simulink model "Kurs"  (R2024a)
settings: Solver=ode1  StartTime=0.0  StopTime=1.2  FixedStep=0.000001  RelTol=1e-3
InitFcn:
  | Kpr = 56;
  | Tpr = 0.002;
  | Rya = 1.78;
  | Tya = 0.16;
  | c = 0.56;
  | J = 0.05;
  | Kot = 0.054;
  | Koc = 0.09;
  | T1 = 0.0013;
  | T2 = 0.0165;
  | T4 = 0.207;
  | K1 = 6.74;
  | K2 = 3.12;
  | K3 = 0.874;
  | X1max = 3;
  | Y2max = 250;
  | Y4max = 90;
  | Z = 17;
  | treg = 0.001;
  | toy = 0.0001;
undefined symbols (not defined in the file or in its folder): Kaw, tre
libraries: slpidlib x5
(part 2 of 2)

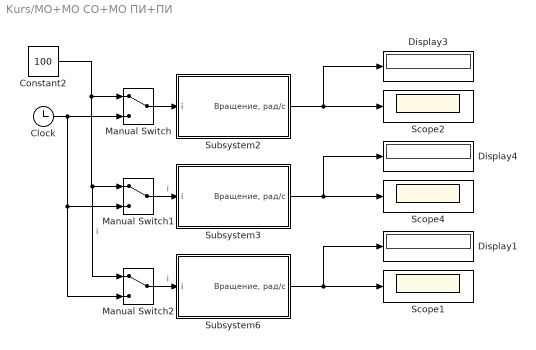
== system Kurs/МО+МО СО+МО ПИ+ПИ ==
  Clock : Clock
  Constant2 : Constant  Value=100
  Display1 : Display
  Display3 : Display
  Display4 : Display
  Manual Switch : ManualSwitch
  Manual Switch1 : ManualSwitch
  Manual Switch2 : ManualSwitch
  Scope1 : Scope
  Scope2 : Scope
  Scope4 : Scope
  Subsystem2 : Subsystem
      mask Display: disp('МО+МО');
  Subsystem3 : Subsystem
      mask Display: disp('СО+МО');
  Subsystem6 : Subsystem  mask{Kpr=Kpr, Tpr=Tpr, Rya=Rya, Tya=Tya, Cm=c, Ce=c, Kot=Kot, Koc=Koc, treg=0.001, toy=Tpr / 100}
      mask prompts: Kpr "Коэффициент усиления преобразователя"; Tpr "Постоянная времени преобразователя"; Rya "Коэффициент усиления тока (1/Rya)"; Tya "Постоянная времени тока"; Cm "Постоянный конструктивный коэффициент (коэффициент связи)"; Ce "Постоянный конструктивный коэффициент (u = Ce*w)"; Kot "Коэффициент обратной связи тока"; Koc "Коэффициент обратной связи угловой скорости"; treg "Шаг дискретизации регуляторов"; toy "Шаг дискретизации ОУ"
      mask Display: disp('ПИ+ПИ');
  wires:
  Subsystem2/1("Вращение, рад/с") -> Display3/1, Scope2/1
  Constant2/1 -> Manual Switch2/1, Manual Switch1/1, Manual Switch/1  "i"
  Subsystem3/1("Вращение, рад/с") -> Display4/1, Scope4/1
  Manual Switch2/1 -> Subsystem6/1(i)  "i"
  Clock/1 -> Manual Switch2/2, Manual Switch1/2, Manual Switch/2
  Subsystem6/1("Вращение, рад/с") -> Display1/1, Scope1/1
  Manual Switch1/1 -> Subsystem3/1(i)  "i"
  Manual Switch/1 -> Subsystem2/1(i)

== system Kurs/МО СО ПИ-регулятор/Subsystem ==
  i : Inport
  1/(rя*(Ts+1)) : TransferFcn  Numerator=[1/Rya]  Denominator=[Tya 1]
  Display : Display
  Gain : Gain  Gain=Tya*Rya/(2*Kpr*Tpr)
  Gain1 : Gain  Gain=1/Tya
  Integrator : Integrator
  Sum : Sum  Inputs=|++
  Sum1 : Sum  Inputs=|+-
  kt/(Ts+1) : TransferFcn  Numerator=[Kpr]  Denominator=[Tpr 1]
  "Ток, А" : Outport
  wires:
  i/1 -> Sum1/1
  kt/(Ts+1)/1 -> 1/(rя*(Ts+1))/1
  Gain1/1 -> Integrator/1
  Gain/1 -> Gain1/1, Display/1, Sum/1
  Integrator/1 -> Sum/2
  1/(rя*(Ts+1))/1 -> "Ток, А"/1, Sum1/2  "Ток, А"
  Sum/1 -> kt/(Ts+1)/1  "U"
  Sum1/1 -> Gain/1  "e(i)"

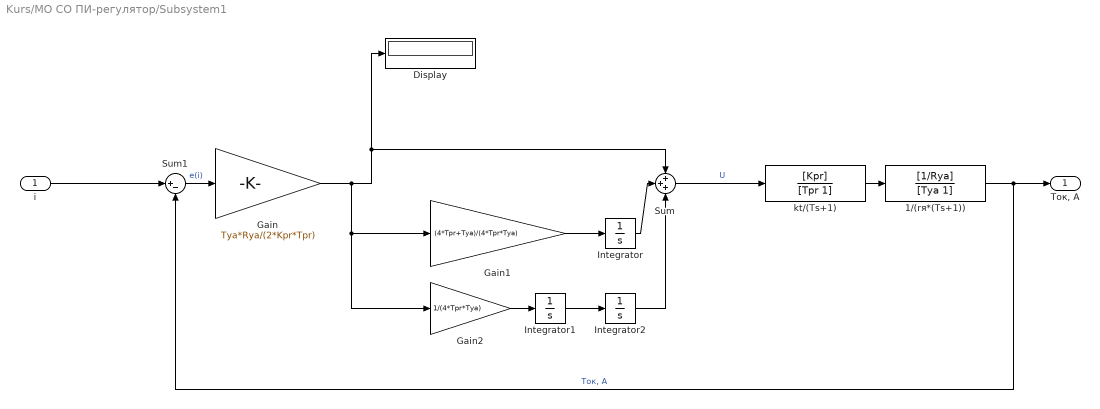
== system Kurs/МО СО ПИ-регулятор/Subsystem1 ==
  i : Inport
  1/(rя*(Ts+1)) : TransferFcn  Numerator=[1/Rya]  Denominator=[Tya 1]
  Display : Display
  Gain : Gain  Gain=Tya*Rya/(2*Kpr*Tpr)
  Gain1 : Gain  Gain=(4*Tpr+Tya)/(4*Tpr*Tya)
  Gain2 : Gain  Gain=1/(4*Tpr*Tya)
  Integrator : Integrator
  Integrator1 : Integrator
  Integrator2 : Integrator
  Sum : Sum  Inputs=+++
  Sum1 : Sum  Inputs=|+-
  kt/(Ts+1) : TransferFcn  Numerator=[Kpr]  Denominator=[Tpr 1]
  "Ток, А" : Outport
  wires:
  i/1 -> Sum1/1
  kt/(Ts+1)/1 -> 1/(rя*(Ts+1))/1
  Gain1/1 -> Integrator/1
  Gain/1 -> Gain2/1, Gain1/1, Display/1, Sum/1
  Integrator/1 -> Sum/2
  1/(rя*(Ts+1))/1 -> "Ток, А"/1, Sum1/2  "Ток, А"
  Sum/1 -> kt/(Ts+1)/1  "U"
  Sum1/1 -> Gain/1  "e(i)"
  Gain2/1 -> Integrator1/1
  Integrator1/1 -> Integrator2/1
  Integrator2/1 -> Sum/3

== system Kurs/МО СО ПИ-регулятор/Subsystem5 ==
  i0(t) : Inport
  1/(rя*(Ts+1)) : TransferFcn  Numerator=[1/Rya]  Denominator=[Tya 1]
  PID Controller9 : slpidlib/PID Controller  Controller=PI  Form=Parallel  TimeDomain=Continuous-time  UseExternalTs=off  SampleTime=treg  IntegratorMethod=Forward Euler  FilterMethod=Forward Euler  ControllerParametersSource=internal  P=0.186679429770122  I=1.09570846442157  UseKiTs=off  D=-544.981619005016  UseExternalDerivativeSource=off  N=0.000737427491300299  UseFilter=on  TunerSelectOption=Transfer Function Based (PID Tuner App)  InitialConditionSource=internal  InitialConditionForIntegrator=0  InitialConditionForFilter=0  DifferentiatorICPrevScaledInput=0  ExternalReset=none  TrackingMode=off  Kt=1  LimitOutput=off  SatLimitsSource=internal  UpperSaturationLimit=12  LowerSaturationLimit=-12  LinearizeAsGain=on  AntiWindupMode=none  Kb=1  LimitIntegrator=off  UpperIntegratorSaturationLimit=inf  LowerIntegratorSaturationLimit=-inf  POutMin=[]  POutMax=[]  IOutMin=[]  IOutMax=[]  DOutMin=[]  DOutMax=[]  NOutMin=[]  NOutMax=[]  SumOutMin=[]  SumOutMax=[]  SaturationOutMin=[]  SaturationOutMax=[]  PParamMin=[]  PParamMax=[]  IParamMin=[]  IParamMax=[]  DParamMin=[]  DParamMax=[]  NParamMin=[]  NParamMax=[]  KbParamMin=[]  KbParamMax=[]  KtParamMin=[]  KtParamMax=[]  KbOutMin=[]  KbOutMax=[]  KtOutMin=[]  KtOutMax=[]  IntegratorOutMin=[]  IntegratorOutMax=[]  FilterOutMin=[]  FilterOutMax=[]  SumI1OutMin=[]  SumI1OutMax=[]  SumI2OutMin=[]  SumI2OutMax=[]  SumI3OutMin=[]  SumI3OutMax=[]  SumI4OutMin=[]  SumI4OutMax=[]  SumDOutMin=[]  SumDOutMax=[]  DifferentiatorOutMin=[]  DifferentiatorOutMax=[]  FilterDiffOutCoefMin=[]  FilterDiffOutCoefMax=[]  ReciprocalOutMin=[]  ReciprocalOutMax=[]  SumDenOutMin=[]  SumDenOutMax=[]  SumNumOutMin=[]  SumNumOutMax=[]  DivideOutMin=[]  DivideOutMax=[]  UdiffTsProdOutMin=[]  UdiffTsProdOutMax=[]  NTsProdOutMin=[]  NTsProdOutMax=[]  UintegralTsProdOutMin=[]  UintegralTsProdOutMax=[]  UngainTsProdOutMin=[]  UngainTsProdOutMax=[]  ClampingZeroOutDataTypeStr=Inherit: Inherit via back propagation  ClampingZeroOutMin=[]  ClampingZeroOutMax=[]  FilterDenConstantOutDataTypeStr=Inherit: Inherit via back propagation  FilterDenConstantOutMin=[]  FilterDenConstantOutMax=[]  PCopyOutDataTypeStr=Inherit: Inherit via back propagation  PCopyOutMin=[]  PCopyOutMax=[]  NCopyOutDataTypeStr=Inherit: Inherit via back propagation  NCopyOutMin=[]  NCopyOutMax=[]  IntegratorContinuousStateAttributes=''  IntegratorStateMustResolveToSignalObject=off  IntegratorRTWStateStorageClass=Auto  FilterContinuousStateAttributes=''  FilterStateMustResolveToSignalObject=off  FilterRTWStateStorageClass=Auto  ParallelPVariant=InternalParameters  IdealPVariant=Disabled  IVariant=InternalParameters  DVariant=Disabled  IntegratorVariant=Continuous  SatVariant=Disabled  AWVariant=Passthrough  PCopyVariant=Disabled  TRVariant=Disabled  FdbkBlocksVariant=Forward  IdealPFdbkVariant=Disabled  SatFdbkVariant=Disabled  DerivativeFilterVariant=Disabled  NVariant=Disabled  NCopyVariant=Disabled_SignalSpec  FilterICVariant=Disabled  IntegratorICVariant=InternalICs  ExternalResetVariant=Disabled  TRSumVariant=Passthrough  SumFdbkVariant=Disabled  SumVariant=Sum_PI  TsampFilterVariant=InternalTs  TsampNgainVariant=Passthrough  TsampIntegralVariant=Disabled_SignalSpec  ExternalSaturationOutDataTypeStr=Inherit: Same as second input  DerivativeSourceVariant=Disabled
  Scope9 : Scope
  Sum16 : Sum  Inputs=|+-
  i(t)1 : Scope
  i(t)3 : Scope
  kt/(Ts+1) : TransferFcn  Numerator=[Kpr]  Denominator=[Tpr 1]
  I(t) : Outport
  wires:
  Sum16/1 -> PID Controller9/1  "e(i)"
  PID Controller9/1 -> Scope9/1, i(t)1/1, kt/(Ts+1)/1  "U"
  i0(t)/1 -> Sum16/1  "i"
  1/(rя*(Ts+1))/1 -> Sum16/2, i(t)3/1, I(t)/1
  kt/(Ts+1)/1 -> 1/(rя*(Ts+1))/1

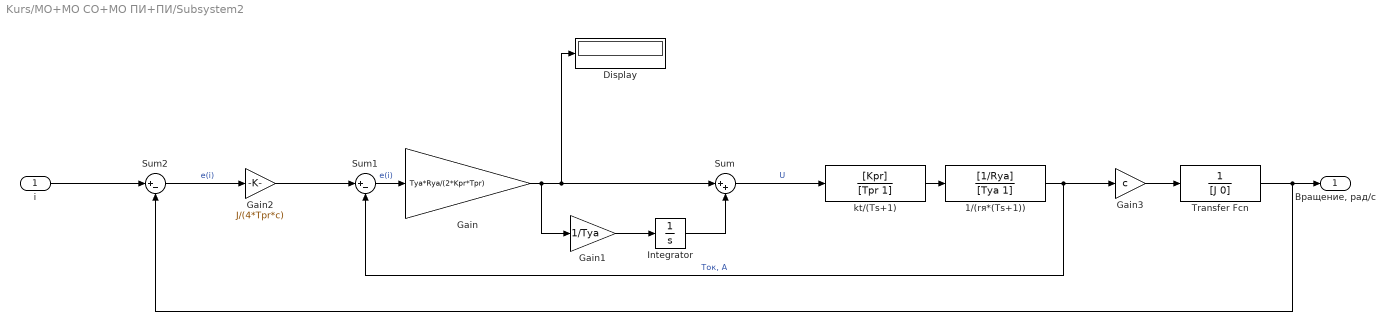
== system Kurs/МО+МО СО+МО ПИ+ПИ/Subsystem2 ==
  i : Inport
  1/(rя*(Ts+1)) : TransferFcn  Numerator=[1/Rya]  Denominator=[Tya 1]
  Display : Display
  Gain : Gain  Gain=Tya*Rya/(2*Kpr*Tpr)
  Gain1 : Gain  Gain=1/Tya
  Gain2 : Gain  Gain=J/(4*Tpr*c)
  Gain3 : Gain  Gain=c
  Integrator : Integrator
  Sum : Sum  Inputs=|++
  Sum1 : Sum  Inputs=|+-
  Sum2 : Sum  Inputs=|+-
  Transfer Fcn : TransferFcn  Denominator=[J 0]
  kt/(Ts+1) : TransferFcn  Numerator=[Kpr]  Denominator=[Tpr 1]
  "Вращение, рад/с" : Outport
  wires:
  kt/(Ts+1)/1 -> 1/(rя*(Ts+1))/1
  Gain1/1 -> Integrator/1
  Gain/1 -> Gain1/1, Display/1, Sum/1
  Integrator/1 -> Sum/2
  1/(rя*(Ts+1))/1 -> Gain3/1, Sum1/2  "Ток, А"
  Sum/1 -> kt/(Ts+1)/1  "U"
  Sum1/1 -> Gain/1  "e(i)"
  Sum2/1 -> Gain2/1  "e(i)"
  Gain2/1 -> Sum1/1
  Gain3/1 -> Transfer Fcn/1
  Transfer Fcn/1 -> Sum2/2, "Вращение, рад/с"/1
  i/1 -> Sum2/1

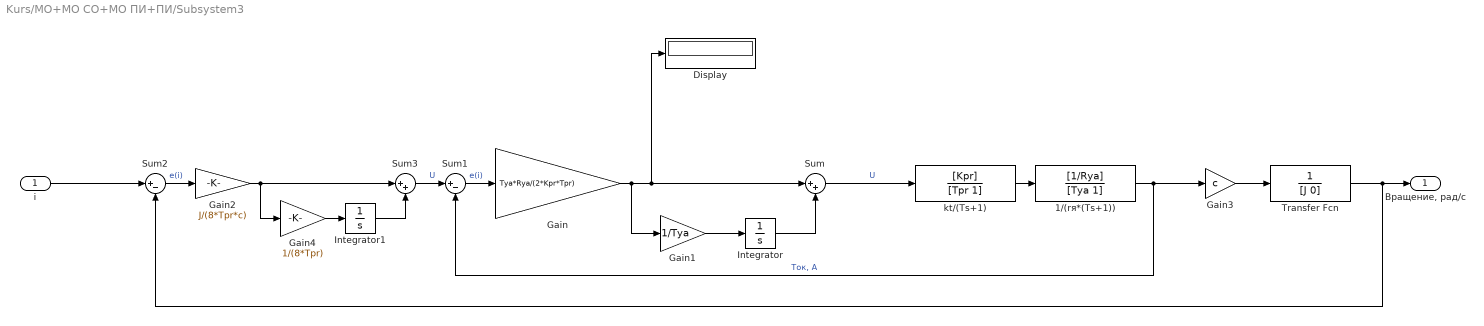
== system Kurs/МО+МО СО+МО ПИ+ПИ/Subsystem3 ==
  i : Inport
  1/(rя*(Ts+1)) : TransferFcn  Numerator=[1/Rya]  Denominator=[Tya 1]
  Display : Display
  Gain : Gain  Gain=Tya*Rya/(2*Kpr*Tpr)
  Gain1 : Gain  Gain=1/Tya
  Gain2 : Gain  Gain=J/(8*Tpr*c)
  Gain3 : Gain  Gain=c
  Gain4 : Gain  Gain=1/(8*Tpr)
  Integrator : Integrator
  Integrator1 : Integrator
  Sum : Sum  Inputs=|++
  Sum1 : Sum  Inputs=|+-
  Sum2 : Sum  Inputs=|+-
  Sum3 : Sum  Inputs=|++
  Transfer Fcn : TransferFcn  Denominator=[J 0]
  kt/(Ts+1) : TransferFcn  Numerator=[Kpr]  Denominator=[Tpr 1]
  "Вращение, рад/с" : Outport
  wires:
  kt/(Ts+1)/1 -> 1/(rя*(Ts+1))/1
  Gain1/1 -> Integrator/1
  Gain/1 -> Gain1/1, Display/1, Sum/1
  Integrator/1 -> Sum/2
  1/(rя*(Ts+1))/1 -> Gain3/1, Sum1/2  "Ток, А"
  Sum/1 -> kt/(Ts+1)/1  "U"
  Sum1/1 -> Gain/1  "e(i)"
  Sum2/1 -> Gain2/1  "e(i)"
  Gain3/1 -> Transfer Fcn/1
  Transfer Fcn/1 -> Sum2/2, "Вращение, рад/с"/1
  i/1 -> Sum2/1
  Sum3/1 -> Sum1/1  "U"
  Integrator1/1 -> Sum3/2
  Gain4/1 -> Integrator1/1
  Gain2/1 -> Gain4/1, Sum3/1

== system Kurs/МО+МО СО+МО ПИ+ПИ/Subsystem6 ==
  i : Inport
  1/(rя*(Ts+1))1 : TransferFcn  Numerator=[1/Rya]  Denominator=[Tya 1]
  Gain3 : Gain  Gain=c
  PID Controller7 : slpidlib/PID Controller  Controller=PI  Form=Ideal  TimeDomain=Continuous-time  UseExternalTs=off  SampleTime=tre  IntegratorMethod=Forward Euler  FilterMethod=Forward Euler  ControllerParametersSource=internal  P=0.143901768144211  I=0.293140363693212  UseKiTs=off  D=30.3034798651177  UseExternalDerivativeSource=off  N=936.857305700604  UseFilter=on  TunerSelectOption=Transfer Function Based (PID Tuner App)  InitialConditionSource=internal  InitialConditionForIntegrator=0  InitialConditionForFilter=0  DifferentiatorICPrevScaledInput=0  ExternalReset=none  TrackingMode=off  Kt=1  LimitOutput=off  SatLimitsSource=internal  UpperSaturationLimit=5  LowerSaturationLimit=-5  LinearizeAsGain=on  AntiWindupMode=none  Kb=1  LimitIntegrator=off  UpperIntegratorSaturationLimit=inf  LowerIntegratorSaturationLimit=-inf  POutMin=[]  POutMax=[]  IOutMin=[]  IOutMax=[]  DOutMin=[]  DOutMax=[]  NOutMin=[]  NOutMax=[]  SumOutMin=[]  SumOutMax=[]  SaturationOutMin=[]  SaturationOutMax=[]  PParamMin=[]  PParamMax=[]  IParamMin=[]  IParamMax=[]  DParamMin=[]  DParamMax=[]  NParamMin=[]  NParamMax=[]  KbParamMin=[]  KbParamMax=[]  KtParamMin=[]  KtParamMax=[]  KbOutMin=[]  KbOutMax=[]  KtOutMin=[]  KtOutMax=[]  IntegratorOutMin=[]  IntegratorOutMax=[]  FilterOutMin=[]  FilterOutMax=[]  SumI1OutMin=[]  SumI1OutMax=[]  SumI2OutMin=[]  SumI2OutMax=[]  SumI3OutMin=[]  SumI3OutMax=[]  SumI4OutMin=[]  SumI4OutMax=[]  SumDOutMin=[]  SumDOutMax=[]  DifferentiatorOutMin=[]  DifferentiatorOutMax=[]  FilterDiffOutCoefMin=[]  FilterDiffOutCoefMax=[]  ReciprocalOutMin=[]  ReciprocalOutMax=[]  SumDenOutMin=[]  SumDenOutMax=[]  SumNumOutMin=[]  SumNumOutMax=[]  DivideOutMin=[]  DivideOutMax=[]  UdiffTsProdOutMin=[]  UdiffTsProdOutMax=[]  NTsProdOutMin=[]  NTsProdOutMax=[]  UintegralTsProdOutMin=[]  UintegralTsProdOutMax=[]  UngainTsProdOutMin=[]  UngainTsProdOutMax=[]  ClampingZeroOutDataTypeStr=Inherit: Inherit via back propagation  ClampingZeroOutMin=[]  ClampingZeroOutMax=[]  FilterDenConstantOutDataTypeStr=Inherit: Inherit via back propagation  FilterDenConstantOutMin=[]  FilterDenConstantOutMax=[]  PCopyOutDataTypeStr=Inherit: Inherit via back propagation  PCopyOutMin=[]  PCopyOutMax=[]  NCopyOutDataTypeStr=Inherit: Inherit via back propagation  NCopyOutMin=[]  NCopyOutMax=[]  IntegratorContinuousStateAttributes=''  IntegratorStateMustResolveToSignalObject=off  IntegratorRTWStateStorageClass=Auto  FilterContinuousStateAttributes=''  FilterStateMustResolveToSignalObject=off  FilterRTWStateStorageClass=Auto  ParallelPVariant=Passthrough  IdealPVariant=InternalParameters  IVariant=InternalParameters  DVariant=Disabled  IntegratorVariant=Continuous  SatVariant=Disabled  AWVariant=Passthrough  PCopyVariant=Disabled  TRVariant=Disabled  FdbkBlocksVariant=Forward  IdealPFdbkVariant=Disabled  SatFdbkVariant=Disabled  DerivativeFilterVariant=Disabled  NVariant=Disabled  NCopyVariant=Disabled_SignalSpec  FilterICVariant=Disabled  IntegratorICVariant=InternalICs  ExternalResetVariant=Disabled  TRSumVariant=Passthrough  SumFdbkVariant=Disabled  SumVariant=Sum_PI  TsampFilterVariant=InternalTs  TsampNgainVariant=Passthrough  TsampIntegralVariant=Disabled_SignalSpec  ExternalSaturationOutDataTypeStr=Inherit: Same as second input  DerivativeSourceVariant=Disabled
  PID Controller9 : slpidlib/PID Controller  Controller=PI  Form=Parallel  TimeDomain=Continuous-time  UseExternalTs=off  SampleTime=treg  IntegratorMethod=Forward Euler  FilterMethod=Forward Euler  ControllerParametersSource=internal  P=0.186679429770122  I=1.09570846442157  UseKiTs=off  D=-544.981619005016  UseExternalDerivativeSource=off  N=0.000737427491300299  UseFilter=on  TunerSelectOption=Transfer Function Based (PID Tuner App)  InitialConditionSource=internal  InitialConditionForIntegrator=0  InitialConditionForFilter=0  DifferentiatorICPrevScaledInput=0  ExternalReset=none  TrackingMode=off  Kt=1  LimitOutput=off  SatLimitsSource=internal  UpperSaturationLimit=12  LowerSaturationLimit=-12  LinearizeAsGain=on  AntiWindupMode=none  Kb=1  LimitIntegrator=off  UpperIntegratorSaturationLimit=inf  LowerIntegratorSaturationLimit=-inf  POutMin=[]  POutMax=[]  IOutMin=[]  IOutMax=[]  DOutMin=[]  DOutMax=[]  NOutMin=[]  NOutMax=[]  SumOutMin=[]  SumOutMax=[]  SaturationOutMin=[]  SaturationOutMax=[]  PParamMin=[]  PParamMax=[]  IParamMin=[]  IParamMax=[]  DParamMin=[]  DParamMax=[]  NParamMin=[]  NParamMax=[]  KbParamMin=[]  KbParamMax=[]  KtParamMin=[]  KtParamMax=[]  KbOutMin=[]  KbOutMax=[]  KtOutMin=[]  KtOutMax=[]  IntegratorOutMin=[]  IntegratorOutMax=[]  FilterOutMin=[]  FilterOutMax=[]  SumI1OutMin=[]  SumI1OutMax=[]  SumI2OutMin=[]  SumI2OutMax=[]  SumI3OutMin=[]  SumI3OutMax=[]  SumI4OutMin=[]  SumI4OutMax=[]  SumDOutMin=[]  SumDOutMax=[]  DifferentiatorOutMin=[]  DifferentiatorOutMax=[]  FilterDiffOutCoefMin=[]  FilterDiffOutCoefMax=[]  ReciprocalOutMin=[]  ReciprocalOutMax=[]  SumDenOutMin=[]  SumDenOutMax=[]  SumNumOutMin=[]  SumNumOutMax=[]  DivideOutMin=[]  DivideOutMax=[]  UdiffTsProdOutMin=[]  UdiffTsProdOutMax=[]  NTsProdOutMin=[]  NTsProdOutMax=[]  UintegralTsProdOutMin=[]  UintegralTsProdOutMax=[]  UngainTsProdOutMin=[]  UngainTsProdOutMax=[]  ClampingZeroOutDataTypeStr=Inherit: Inherit via back propagation  ClampingZeroOutMin=[]  ClampingZeroOutMax=[]  FilterDenConstantOutDataTypeStr=Inherit: Inherit via back propagation  FilterDenConstantOutMin=[]  FilterDenConstantOutMax=[]  PCopyOutDataTypeStr=Inherit: Inherit via back propagation  PCopyOutMin=[]  PCopyOutMax=[]  NCopyOutDataTypeStr=Inherit: Inherit via back propagation  NCopyOutMin=[]  NCopyOutMax=[]  IntegratorContinuousStateAttributes=''  IntegratorStateMustResolveToSignalObject=off  IntegratorRTWStateStorageClass=Auto  FilterContinuousStateAttributes=''  FilterStateMustResolveToSignalObject=off  FilterRTWStateStorageClass=Auto  ParallelPVariant=InternalParameters  IdealPVariant=Disabled  IVariant=InternalParameters  DVariant=Disabled  IntegratorVariant=Continuous  SatVariant=Disabled  AWVariant=Passthrough  PCopyVariant=Disabled  TRVariant=Disabled  FdbkBlocksVariant=Forward  IdealPFdbkVariant=Disabled  SatFdbkVariant=Disabled  DerivativeFilterVariant=Disabled  NVariant=Disabled  NCopyVariant=Disabled_SignalSpec  FilterICVariant=Disabled  IntegratorICVariant=InternalICs  ExternalResetVariant=Disabled  TRSumVariant=Passthrough  SumFdbkVariant=Disabled  SumVariant=Sum_PI  TsampFilterVariant=InternalTs  TsampNgainVariant=Passthrough  TsampIntegralVariant=Disabled_SignalSpec  ExternalSaturationOutDataTypeStr=Inherit: Same as second input  DerivativeSourceVariant=Disabled
  Sum1 : Sum  Inputs=|+-
  Sum2 : Sum  Inputs=|+-
  Transfer Fcn : TransferFcn  Denominator=[J 0]
  kt/(Ts+1)1 : TransferFcn  Numerator=[Kpr]  Denominator=[Tpr 1]
  "Вращение, рад/с" : Outport
  wires:
  Sum2/1 -> PID Controller7/1  "e(i)"
  Transfer Fcn/1 -> Sum2/2, "Вращение, рад/с"/1
  PID Controller9/1 -> kt/(Ts+1)1/1  "U"
  1/(rя*(Ts+1))1/1 -> Gain3/1, Sum1/2  "Ток, А"
  kt/(Ts+1)1/1 -> 1/(rя*(Ts+1))1/1
  Gain3/1 -> Transfer Fcn/1
  i/1 -> Sum2/1
  Sum1/1 -> PID Controller9/1  "e(i)"
  PID Controller7/1 -> Sum1/1  "U"

== stateflow chart Kurs/Subsystem4/Chart1 ==
  (default) -> (junction 7)
  (junction 7) -> (junction 9) : {k1 = (k * dt)/(T+dt);
      | k2 = T/(T+dt);
      | y = k1 * x + k2 * y_pr;}
  (junction 9) -> (junction 10) : {y_pr = y;}
  data: k input double; T input double; dt input double; x input double; y output double; y_pr local double; k1 output double; k2 output double

== stateflow chart Kurs/Subsystem4/Chart3 ==
  (default) -> (junction 7)
  (junction 7) -> (junction 9) : {k1 = (k * dt)/(T+dt);
      | k2 = T/(T+dt);
      | y = k1 * x + k2 * y_pr;}
  (junction 9) -> (junction 10) : {y_pr = y;}
  data: k input double; T input double; dt input double; x input double; y output double; y_pr local double; k1 output double; k2 output double

== stateflow chart Kurs/Subsystem1/Chart2 ==
  (default) -> (junction 7)
  (junction 7) -> (junction 9) : {k1 = dt/Tu;
      | y = y_pr + Kp * (err - err_pr + dt/Tu * err);}
  (junction 9) -> (junction 10) : {y_pr = y;
      | err_pr = err;}
  data: Kp input double; Tu input double; dt input double; err input double; y output double; y_pr local double; err_pr local double; k1 local double

== stateflow chart Kurs/Subsystem1/Chart3 ==
  (default) -> (junction 7)
  (junction 7) -> (junction 9) : {k1 = (k * dt)/(T+dt);
      | k2 = T/(T+dt);
      | y = k1 * x + k2 * y_pr;}
  (junction 9) -> (junction 10) : {y_pr = y;}
  data: k input double; T input double; dt input double; x input double; y output double; y_pr local double; k1 output double; k2 output double

== stateflow chart Kurs/Subsystem6/Chart1 ==
  (default) -> (junction 7)
  (junction 7) -> (junction 9) : {k1 = (k * dt)/(T+dt);
      | k2 = T/(T+dt);
      | y = k1 * x + k2 * y_pr;}
  (junction 9) -> (junction 10) : {y_pr = y;}
  data: k input double; T input double; dt input double; x input double; y output double; y_pr local double; k1 local double; k2 local double

== stateflow chart Kurs/Subsystem2/Chart3 ==
  (default) -> (junction 7)
  (junction 7) -> (junction 9) : {k1 = (k * dt)/(T+dt);
      | k2 = T/(T+dt);
      | y = k1 * x + k2 * y_pr;}
  (junction 9) -> (junction 10) : {y_pr = y;}
  data: k input double; T input double; dt input double; x input double; y output double; y_pr local double; k1 output double; k2 output double

== stateflow chart Kurs/Subsystem2/Chart4 ==
  (default) -> (junction 7)
  (junction 7) -> (junction 9) : {y = y_pr + Kp * (err - err_pr + dt/Tu * err);}
  (junction 9) -> (junction 10) : {y_pr = y;
      | err_pr = err;}
  data: Kp input double; Tu input double; dt input double; err input double; y output double; y_pr local double; err_pr local double

== stateflow chart Kurs/Subsystem6/Chart2 ==
  (default) -> (junction 7)
  (junction 7) -> (junction 9) : {k1 = dt/Tu;
      | y = y_pr + Kp * (err - err_pr + dt/Tu * err);}
  (junction 9) -> (junction 10) : {y_pr = y;
      | err_pr = err;}
  data: Kp input double; Tu input double; dt input double; err input double; y output double; y_pr local double; err_pr local double; k1 local double

== stateflow chart Kurs/Subsystem6/Chart3 ==
  (default) -> (junction 7)
  (junction 7) -> (junction 9) : {k1 = dt/Tu;
      | y = y_pr + Kp * (err - err_pr + k1 * err);}
  (junction 9) -> (junction 10) : {y_pr = y;
      | err_pr = err;}
  data: Kp input double; Tu input double; dt input double; err input double; y output double; y_pr local double; err_pr local double; k1 local double

== stateflow chart Kurs/Subsystem6/Chart4 ==
  (default) -> (junction 7)
  (junction 7) -> (junction 9) : {k1 = (k * dt)/(T+dt);
      | k2 = T/(T+dt);
      | y = k1 * x + k2 * y_pr;}
  (junction 9) -> (junction 10) : {y_pr = y;}
  data: k input double; T input double; dt input double; x input double; y output double; y_pr local double; k1 local double; k2 local double

== stateflow chart Kurs/Subsystem6/Chart5 ==
  (default) -> (junction 7)
  (junction 7) -> (junction 9) : {k1 = dt/T;
      | y = k1 * x + y_pr;}
  (junction 9) -> (junction 10) : {y_pr = y;}
  data: T input double; dt input double; x input double; y output double; y_pr local double; k1 local double

== stateflow chart Kurs/Chart2 ==
  (default) -> (junction 7)
  (junction 7) -> (junction 9) : {k1 = (k * dt)/(T+dt);
      | k2 = T/(T+dt);
      | y = k1 * x + k2 * y_pr;}
  (junction 9) -> (junction 10) : {y_pr = y;}
  data: k input double; T input double; dt input double; x input double; y output double; y_pr local double; k1 local double; k2 local double

== stateflow chart Kurs/Subsystem7/Chart1 ==
  (default) -> (junction 7)
  (junction 7) -> (junction 9) : {k1 = (k * dt)/(T+dt);
      | k2 = T/(T+dt);
      | y = k1 * x + k2 * y_pr;}
  (junction 9) -> (junction 10) : {y_pr = y;}
  data: k input double; T input double; dt input double; x input double; y output double; y_pr local double; k1 local double; k2 local double

== stateflow chart Kurs/Subsystem7/Chart2 ==
  (default) -> (junction 7)
  (junction 7) -> (junction 9) : {k1 = dt/Tu;
      | y = OFF * (y_pr + Kp * (err - err_pr + dt/Tu * err));}
  (junction 9) -> (junction 10) : {y_pr = y;
      | err_pr = err;}
  data: Kp input double; Tu input double; dt input double; err input double; y output double; y_pr local double; err_pr local double; k1 local double; OFF input double

== stateflow chart Kurs/Chart4 ==
  (default) -> (junction 7)
  (junction 7) -> (junction 9) : {k1 = (k * dt)/(T+dt);
      | k2 = T/(T+dt);
      | y = k1 * x + k2 * y_pr;}
  (junction 9) -> (junction 10) : {y_pr = y;}
  data: k input double; T input double; dt input double; x input double; y output double; y_pr local double; k1 local double; k2 local double

== stateflow chart Kurs/Subsystem7/Chart4 ==
  (default) -> (junction 7)
  (junction 7) -> (junction 9) : {k1 = (k * dt)/(T+dt);
      | k2 = T/(T+dt);
      | y = k1 * x + k2 * y_pr;}
  (junction 9) -> (junction 10) : {y_pr = y;}
  data: k input double; T input double; dt input double; x input double; y output double; y_pr local double; k1 local double; k2 local double

== stateflow chart Kurs/Subsystem7/Chart5 ==
  (default) -> (junction 7)
  (junction 7) -> (junction 9) : {k1 = dt/T;
      | y = k1 * x + y_pr;}
  (junction 9) -> (junction 10) : {y_pr = y;}
  data: T input double; dt input double; x input double; y output double; y_pr local double; k1 local double

== stateflow chart Kurs/Subsystem7/Chart6 ==
  (default) -> (junction 7)
  (junction 7) -> (junction 9) : {k1 = dt/Tu;
      | Prop = Kp * err;
      | Int_ = OFF * (Int + Prop * k1 + Kaw * ErrSat * k1);
      | y = OFF * (Prop + Int_);}
  (junction 9) -> (junction 26) : {Int = Int_;}
  data: Kp input double; Tu input double; dt input double; err input double; y output double; Int local double; k1 local double; ErrSat input double; Kaw input double; Int_ local double; Prop local double; err_pr local double; OFF input double

== stateflow chart Kurs/Chart5 ==
  (default) -> (junction 7)
  (junction 7) -> (junction 9) : {k1 = dt/T;
      | y = k1 * x + y_pr;}
  (junction 9) -> (junction 10) : {y_pr = y;}
  data: T input double; dt input double; x input double; y output double; y_pr local double; k1 local double

== stateflow chart Kurs/Chart6 ==
  (default) -> (junction 7)
  (junction 7) -> (junction 9) : {k1 = dt/Tu;
      | Prop = Kp * err;
      | Int_ = Int + Prop * k1 + Kaw * ErrSat * k1;
      | y = Prop + Int_;}
  (junction 9) -> (junction 26) : {Int = Int_;}
  data: Kp input double; Tu input double; dt input double; err input double; y output double; Int local double; k1 local double; ErrSat input double; Kaw input double; Int_ local double; Prop local double

== stateflow chart Kurs/Chart1 ==
  (default) -> (junction 7)
  (junction 7) -> (junction 9) : {k1 = dt/Tu;
      | Prop = Kp * err;
      | Int_ = Int + Prop * k1;
      | y = Prop + Int_;}
  (junction 9) -> (junction 26) : {Int = Int_;}
  data: Kp input double; Tu input double; dt input double; err input double; y output double; Int local double; k1 local double; Int_ local double; Prop local double

== stateflow chart Kurs/Chart3 ==
  (default) -> (junction 7)
  (junction 7) -> (junction 9) : {k1 = dt/Tu;
      | y = y_pr + Kp * (err - err_pr + dt/Tu * err);}
  (junction 9) -> (junction 10) : {y_pr = y;
      | err_pr = err;}
  data: Kp input double; Tu input double; dt input double; err input double; y output double; y_pr local double; err_pr local double; k1 local double

== stateflow chart Kurs/Chart7 ==
  (default) -> (junction 7)
  (junction 7) -> (junction 9) : {k1 = dt/Tu;
      | y = y_pr + Kp * (err - err_pr + k1 * err);}
  (junction 9) -> (junction 10) : {y_pr = y;
      | err_pr = err;}
  data: Kp input double; Tu input double; dt input double; err input double; y output double; y_pr local double; err_pr local double; k1 local double

== stateflow chart Kurs/Chart8 ==
  (default) -> (junction 7)
  (junction 7) -> (junction 9) : {k1 = (k * dt)/(T+dt);
      | k2 = T/(T+dt);
      | y = k1 * x + k2 * y_pr;}
  (junction 9) -> (junction 10) : {y_pr = y;}
  data: k input double; T input double; dt input double; x input double; y output double; y_pr local double; k1 local double; k2 local double

== stateflow chart Kurs/Chart9 ==
  (default) -> (junction 7)
  (junction 7) -> (junction 9) : {k1 = dt/T;
      | y = k1 * x + y_pr;}
  (junction 9) -> (junction 10) : {y_pr = y;}
  data: T input double; dt input double; x input double; y output double; y_pr local double; k1 local double

== stateflow chart Kurs/Subsystem7/Chart3 ==
  (default) -> (junction 38)
  (junction 38) -> (junction 56) [order 2] : [y < Ymin]
  (junction 38) -> (junction 54) [order 1] : [y > Ymax]
  (junction 38) -> (junction 62) [order 3] : [y <= Ymax || y >= Ymin]
  (junction 54) -> (junction 58) : {y_lim = Ymax;
      | flag = 1;}
  (junction 62) -> (junction 64) : {y_lim = y;
      | ErrSat = 0;
      | flag = 3;}
  (junction 56) -> (junction 60) : {y_lim = Ymin;
      | flag = 2;}
  (junction 58) -> (junction 66) : {ErrSat = y_lim - y;}
  (junction 64) -> (junction 69) : {flag = 4;}
  (junction 60) -> (junction 66) : {ErrSat = y_lim - y;}
  (junction 66) -> (junction 69) : {flag = 4;}
  data: Ymax input double; y input double; y_lim output double; flag local double; ErrSat output double; Ymin input double

== stateflow chart Kurs/Chart10 ==
  (default) -> (junction 38)
  (junction 38) -> (junction 56) [order 2] : [y < Ymin]
  (junction 38) -> (junction 54) [order 1] : [y > Ymax]
  (junction 38) -> (junction 62) [order 3] : [y <= Ymax || y >= Ymin]
  (junction 54) -> (junction 58) : {y_lim = Ymax;
      | flag = 1;}
  (junction 62) -> (junction 64) : {y_lim = y;
      | ErrSat = 0;
      | flag = 3;}
  (junction 56) -> (junction 60) : {y_lim = Ymax;
      | flag = 2;}
  (junction 58) -> (junction 66) : {ErrSat = y_lim - y;}
  (junction 60) -> (junction 66) : {ErrSat = y_lim - y;}
  (junction 64) -> (junction 69) : {flag = 4;}
  (junction 66) -> (junction 69) : {flag = 4;}
  data: Ymax input double; y input double; y_lim output double; flag local double; ErrSat output double; Ymin input double

== stateflow chart Kurs/Chart11 ==
  (default) -> (junction 38)
  (junction 38) -> (junction 56) [order 2] : [y < Ymin]
  (junction 38) -> (junction 54) [order 1] : [y > Ymax]
  (junction 38) -> (junction 62) [order 3] : [y <= Ymax || y >= Ymin]
  (junction 54) -> (junction 58) : {y_lim = Ymax;
      | flag = 1;}
  (junction 62) -> (junction 64) : {y_lim = y;
      | ErrSat = 0;
      | flag = 3;}
  (junction 56) -> (junction 60) : {y_lim = Ymax;
      | flag = 2;}
  (junction 58) -> (junction 66) : {ErrSat = y_lim - y;}
  (junction 60) -> (junction 66) : {ErrSat = y_lim - y;}
  (junction 64) -> (junction 69) : {flag = 4;}
  (junction 66) -> (junction 69) : {flag = 4;}
  data: Ymax input double; y input double; y_lim output double; flag local double; ErrSat output double; Ymin input double

== stateflow chart Kurs/Subsystem7/Chart7 ==
  (default) -> (junction 38)
  (junction 38) -> (junction 56) [order 2] : [y < Ymin]
  (junction 38) -> (junction 54) [order 1] : [y > Ymax]
  (junction 38) -> (junction 62) [order 3] : [y <= Ymax || y >= Ymin]
  (junction 54) -> (junction 58) : {y_lim = Ymax;
      | flag = 1;}
  (junction 62) -> (junction 64) : {y_lim = y;
      | ErrSat = 0;
      | flag = 3;}
  (junction 56) -> (junction 60) : {y_lim = Ymin;
      | flag = 2;}
  (junction 58) -> (junction 66) : {ErrSat = y_lim - y;}
  (junction 64) -> (junction 69) : {flag = 4;}
  (junction 60) -> (junction 66) : {ErrSat = y_lim - y;}
  (junction 66) -> (junction 69) : {flag = 4;}
  data: Ymax input double; y input double; y_lim output double; flag local double; ErrSat output double; Ymin input double

== stateflow chart Kurs/Subsystem7/Chart8 ==
  (default) -> (junction 38)
  (junction 38) -> (junction 56) [order 2] : [y < Ymin]
  (junction 38) -> (junction 54) [order 1] : [y > Ymax]
  (junction 38) -> (junction 62) [order 3] : [y <= Ymax || y >= Ymin]
  (junction 54) -> (junction 58) : {y_lim = Ymax;
      | flag = 1;}
  (junction 62) -> (junction 64) : {y_lim = y;
      | ErrSat = 0;
      | flag = 3;}
  (junction 56) -> (junction 60) : {y_lim = Ymin;
      | flag = 2;}
  (junction 58) -> (junction 66) : {ErrSat = y_lim - y;}
  (junction 64) -> (junction 69) : {flag = 4;}
  (junction 60) -> (junction 66) : {ErrSat = y_lim - y;}
  (junction 66) -> (junction 69) : {flag = 4;}
  data: Ymax input double; y input double; y_lim output double; flag local double; ErrSat output double; Ymin input double

== stateflow chart Kurs/Chart ==
  state INIT_STATE
    red_l=0;
    blue_l=0;
    green_l=0;
    error=0;
    X1=0;
    counter=0;
    t_st=0;
    T_pr=0;
  state CRIT_OBJ
    t_st = t;
  state ON
    X1=1;
  state ERR_OBJ
    error = 1;
    X1 = 0;
    red_l=0;
    blue_l=0;
    green_l=0;
  state RED_ERR_ON
    red_l=1;
  state RED_ERR_OFF
    red_l=0;
    counter = 0;
  state NORM_STATE
    t_st = 0;
  state DOOR_OPEN
    red_l=0;
    blue_l=1;
    green_l=1;
  state HOT_STATE
    red_l=1;
    blue_l=0;
    green_l=0;
    T_pr=T;
  state COLD_STATE
    red_l=0;
    blue_l=1;
    green_l=0;
    T_pr=T;
  state TEMP_STATE
    red_l=0;
    blue_l=0;
    green_l=1;
    T_pr=T;
  RED_ERR_OFF -> INIT_STATE [order 2] : [on == 0]
  (default) -> INIT_STATE
  RED_ERR_ON -> INIT_STATE [order 2] : [on == 0]
  ERR_OBJ -> INIT_STATE [order 2] : [on == 0]
  ON -> INIT_STATE [order 2] : [on == 0]
  ON -> CRIT_OBJ [order 1] : [(T >= Tmax || T <= Tmin) && t_st == 0]
  CRIT_OBJ -> ON
  INIT_STATE -> ON : [on == 1]
  RED_ERR_ON -> (junction 17) [order 1]
  ON -> ERR_OBJ [order 3] : [(T >= Tmax || T <= Tmin) && (t - t_st) >= 0.5]
  ON -> NORM_STATE [order 4] : [(T < Tmax || T > Tmin) && t_st == 0 && t_st == 0 && after(0.005,sec)]
  DOOR_OPEN -> ON
  HOT_STATE -> ON : [after(0.005,sec)]
  COLD_STATE -> ON : [after(0.005,sec)]
  TEMP_STATE -> ON : [after(0.005,sec)]
  (junction 22) -> RED_ERR_ON [order 1] : [counter >= 500 && counter < 1000]
  (junction 17) -> (junction 22) : {counter = counter + 1;}
  ERR_OBJ -> (junction 17) [order 1]
  (junction 22) -> ERR_OBJ [order 3] : [counter < 500]
  (junction 22) -> RED_ERR_OFF [order 2] : [counter >= 1000 && red_l == 1]
  RED_ERR_OFF -> (junction 17) [order 1]
  NORM_STATE -> TEMP_STATE [order 4] : [Z == 0 && (abs(T - T_pr) < T_dz) && (abs(T - Tset) < 0.05) && after(0.005,sec)]
  NORM_STATE -> COLD_STATE [order 3] : [Z == 0 && (abs(T - T_pr) > T_dz) && after(0.005,sec)]
  NORM_STATE -> HOT_STATE [order 2] : [Z == 0 && (T - T_pr > T_dz) && after(0.005,sec)]
  NORM_STATE -> DOOR_OPEN [order 1] : [Z > 0 && after(0.005,sec)]
  data: counter local; t_st local; red_l output; blue_l output; green_l output; error output; X1 output; t input size=1; Tmin input size=1; Tmax input size=1; T input size=1; T_dz input size=1; Z input size=1; on input size=1; T_pr local; Tset input size=1

== stateflow chart Kurs/Subsystem7/Chart ==
  state INIT_STATE
    red_l=0;
    blue_l=0;
    green_l=0;
    error=0;
    X1=0;
    counter=0;
    t_st=0;
    T_pr=0;
  state CRIT_OBJ
    t_st = t;
  state ON
    X1=1;
  state ERR_OBJ
    error = 1;
    X1 = 0;
    red_l=0;
    blue_l=0;
    green_l=0;
  state RED_ERR_ON
    red_l=1;
  state RED_ERR_OFF
    red_l=0;
    counter = 0;
  state NORM_STATE
    t_st = 0;
  state DOOR_OPEN
    red_l=0;
    blue_l=1;
    green_l=1;
  state HOT_STATE
    red_l=1;
    blue_l=0;
    green_l=0;
    T_pr=T;
  state COLD_STATE
    red_l=0;
    blue_l=1;
    green_l=0;
    T_pr=T;
  state TEMP_STATE
    red_l=0;
    blue_l=0;
    green_l=1;
    T_pr=T;
  RED_ERR_OFF -> INIT_STATE [order 2] : [on == 0]
  RED_ERR_ON -> INIT_STATE [order 2] : [on == 0]
  (default) -> INIT_STATE
  ERR_OBJ -> INIT_STATE [order 2] : [on == 0]
  RED_ERR_ON -> (junction 17) [order 1]
  ON -> INIT_STATE [order 2] : [on == 0]
  ON -> CRIT_OBJ [order 1] : [(T >= Tmax || T <= Tmin) && t_st == 0]
  INIT_STATE -> ON : [on == 1]
  CRIT_OBJ -> ON
  ON -> ERR_OBJ [order 3] : [(T >= Tmax || T <= Tmin) && (t - t_st) >= 0.5]
  ON -> NORM_STATE [order 4] : [(T < Tmax || T > Tmin) && (t - t_st) < 0.5 && t_st == 0]
  DOOR_OPEN -> ON
  HOT_STATE -> ON
  COLD_STATE -> ON
  TEMP_STATE -> ON
  (junction 22) -> RED_ERR_ON [order 1] : [counter >= 50000 && counter < 100000]
  (junction 17) -> (junction 22) : {counter = counter + 1;}
  ERR_OBJ -> (junction 17) [order 1]
  (junction 22) -> ERR_OBJ [order 3] : [counter < 50000]
  (junction 22) -> RED_ERR_OFF [order 2] : [counter >= 100000 && red_l == 1]
  RED_ERR_OFF -> (junction 17) [order 1]
  NORM_STATE -> TEMP_STATE [order 4] : [Z == 0 && (abs(T - T_pr) < T_dz) && (abs(T - Tset) < 0.05) && after(0.005,sec)]
  NORM_STATE -> COLD_STATE [order 3] : [Z == 0 && (abs(T - T_pr) > T_dz) && after(0.005,sec)]
  NORM_STATE -> HOT_STATE [order 2] : [Z == 0 && (T - T_pr > T_dz) && after(0.005,sec)]
  NORM_STATE -> DOOR_OPEN [order 1] : [Z > 0]
  data: counter local; t_st local; red_l output; blue_l output; green_l output; error output; X1 output; t input size=1; Tmin input size=1; Tmax input size=1; T input size=1; T_dz input size=1; Z input size=1; on input size=1; T_pr local; Tset input size=1

== stateflow chart Kurs/Subsystem2/Chart1 ==
  (default) -> (junction 7)
  (junction 7) -> (junction 9) : {k1 = (k * dt)/(T+dt);
      | k2 = T/(T+dt);
      | y = k1 * x + k2 * y_pr;}
  (junction 9) -> (junction 10) : {y_pr = y;}
  data: k input double; T input double; dt input double; x input double; y output double; y_pr local double; k1 output double; k2 output double

== stateflow chart Kurs/Chart12 ==
  (default) -> (junction 7)
  (junction 7) -> (junction 9) : {k1 = (k * dt)/(T+dt);
      | k2 = T/(T+dt);
      | y = k1 * x + k2 * y_pr;}
  (junction 9) -> (junction 10) : {y_pr = y;}
  data: k input double; T input double; dt input double; x input double; y output double; y_pr local double; k1 local double; k2 local double

== stateflow chart Kurs/Chart13 ==
  (default) -> (junction 7)
  (junction 7) -> (junction 9) : {k1 = dt/T;
      | y = k1 * x + y_pr;}
  (junction 9) -> (junction 10) : {y_pr = y;}
  data: T input double; dt input double; x input double; y output double; y_pr local double; k1 local double

== stateflow chart Kurs/Chart14 ==
  (default) -> (junction 38)
  (junction 38) -> (junction 56) [order 2] : [y < Ymin]
  (junction 38) -> (junction 54) [order 1] : [y > Ymax]
  (junction 38) -> (junction 62) [order 3] : [y <= Ymax || y >= Ymin]
  (junction 54) -> (junction 58) : {y_lim = Ymax;
      | flag = 1;}
  (junction 62) -> (junction 64) : {y_lim = y;
      | ErrSat = 0;
      | flag = 3;}
  (junction 56) -> (junction 60) : {y_lim = Ymin;
      | flag = 2;}
  (junction 58) -> (junction 66) : {ErrSat = y_lim - y;}
  (junction 64) -> (junction 69) : {flag = 4;}
  (junction 60) -> (junction 66) : {ErrSat = y_lim - y;}
  (junction 66) -> (junction 69) : {flag = 4;}
  data: Ymax input double; y input double; y_lim output double; flag local double; ErrSat output double; Ymin input double

== stateflow chart Kurs/Chart15 ==
  (default) -> (junction 7)
  (junction 7) -> (junction 9) : {k1 = (k * dt)/(T+dt);
      | k2 = T/(T+dt);
      | y = k1 * x + k2 * y_pr;}
  (junction 9) -> (junction 10) : {y_pr = y;}
  data: k input double; T input double; dt input double; x input double; y output double; y_pr local double; k1 local double; k2 local double

== stateflow chart Kurs/Chart16 ==
  (default) -> (junction 7)
  (junction 7) -> (junction 9) : {k1 = dt/T;
      | y = k1 * x + y_pr;}
  (junction 9) -> (junction 10) : {y_pr = y;}
  data: T input double; dt input double; x input double; y output double; y_pr local double; k1 local double

== stateflow chart Kurs/Chart17 ==
  (default) -> (junction 7)
  (junction 7) -> (junction 9) : {k1 = dt/Tu;
      | Prop = Kp * err;
      | Int_ = OFF * (Int + Prop * k1 + Kaw * ErrSat * k1);
      | y = OFF * (Prop + Int_);}
  (junction 9) -> (junction 26) : {Int = Int_;}
  data: Kp input double; Tu input double; dt input double; err input double; y output double; Int local double; k1 local double; ErrSat input double; Kaw input double; Int_ local double; Prop local double; err_pr local double; OFF input double

== stateflow chart Kurs/Chart18 ==
  (default) -> (junction 38)
  (junction 38) -> (junction 56) [order 2] : [y < Ymin]
  (junction 38) -> (junction 54) [order 1] : [y > Ymax]
  (junction 38) -> (junction 62) [order 3] : [y <= Ymax || y >= Ymin]
  (junction 54) -> (junction 58) : {y_lim = Ymax;
      | flag = 1;}
  (junction 62) -> (junction 64) : {y_lim = y;
      | ErrSat = 0;
      | flag = 3;}
  (junction 56) -> (junction 60) : {y_lim = Ymin;
      | flag = 2;}
  (junction 58) -> (junction 66) : {ErrSat = y_lim - y;}
  (junction 64) -> (junction 69) : {flag = 4;}
  (junction 60) -> (junction 66) : {ErrSat = y_lim - y;}
  (junction 66) -> (junction 69) : {flag = 4;}
  data: Ymax input double; y input double; y_lim output double; flag local double; ErrSat output double; Ymin input double

== stateflow chart Kurs/Subsystem1/Chart1 ==
  (default) -> (junction 7)
  (junction 7) -> (junction 9) : {k1 = (k * dt)/(T+dt);
      | k2 = T/(T+dt);
      | y = k1 * x + k2 * y_pr;}
  (junction 9) -> (junction 10) : {y_pr = y;}
  data: k input double; T input double; dt input double; x input double; y output double; y_pr local double; k1 output double; k2 output double

== stateflow chart Kurs/Chart19 ==
  (default) -> (junction 38)
  (junction 38) -> (junction 56) [order 2] : [y < Ymin]
  (junction 38) -> (junction 54) [order 1] : [y > Ymax]
  (junction 38) -> (junction 62) [order 3] : [y <= Ymax || y >= Ymin]
  (junction 54) -> (junction 58) : {y_lim = Ymax;
      | flag = 1;}
  (junction 62) -> (junction 64) : {y_lim = y;
      | ErrSat = 0;
      | flag = 3;}
  (junction 56) -> (junction 60) : {y_lim = Ymin;
      | flag = 2;}
  (junction 58) -> (junction 66) : {ErrSat = y_lim - y;}
  (junction 64) -> (junction 69) : {flag = 4;}
  (junction 60) -> (junction 66) : {ErrSat = y_lim - y;}
  (junction 66) -> (junction 69) : {flag = 4;}
  data: Ymax input double; y input double; y_lim output double; flag local double; ErrSat output double; Ymin input double

== stateflow chart Kurs/Chart20 ==
  (default) -> (junction 7)
  (junction 7) -> (junction 9) : {k1 = dt/Tu;
      | Prop = Kp * err;
      | Int_ = OFF * (Int + Prop * k1);
      | y = OFF * (Prop + Int_);}
  (junction 9) -> (junction 26) : {Int = Int_;}
  data: Kp input double; Tu input double; dt input double; err input double; y output double; Int local double; k1 local double; Int_ local double; Prop local double; err_pr local double; OFF input double
